simulink model "A5Q3"  (R2017a)
settings: Solver=VariableStepAuto  StartTime=0.0  StopTime=300  MaxStep=0.001  RelTol=1e-3
values from neighbouring files (symbols this model uses):
  alpha_dc = alpha_c/20    (= 0.349219619187)    [Project5Var.m]
  alpha_f = 5*alpha_p    (= 3.49219619187)    [Project5Var.m]
  alpha_fc = 0.5*alpha_c    (= 3.49219619187)    [Project5Var.m]
  C = 1.5*1800/1000*80*10^-6 * Z_base *w_base    (= 1.1558539944)    [Project5Var.m]
  E = 1.0    (= 1)    [Project5Var.m]
  I_base = 1    [Project5Var.m]
  K = sqrt(3/2)    [Project5Var.m]
  ki = alpha_c*(R+Ra)    (= 11.8344493889)    [Project5Var.m]
  ki_dc = alpha_dc^2/2    (= 0.0609771712125)    [Project5Var.m]
  ki_pll = alpha_p^2/2    (= 0.24390868485)    [Project5Var.m]
  kp = alpha_c*Lsigma    (= 1.69441359229)    [Project5Var.m]
  kp_dc = alpha_dc    (= 0.349219619187)    [Project5Var.m]
  kp_pll = alpha_p    (= 0.698439238374)    [Project5Var.m]
  Lsigma = 0.2426    [Project5Var.m]
  Ra = alpha_c*Lsigma-R    (= 1.58785359229)    [Project5Var.m]
  V_base = 1    [Project5Var.m]
  wref = 1.0    (= 1)    [Project5Var.m]
settings Model: Creator=Oskar  LastModifiedBy=Callum

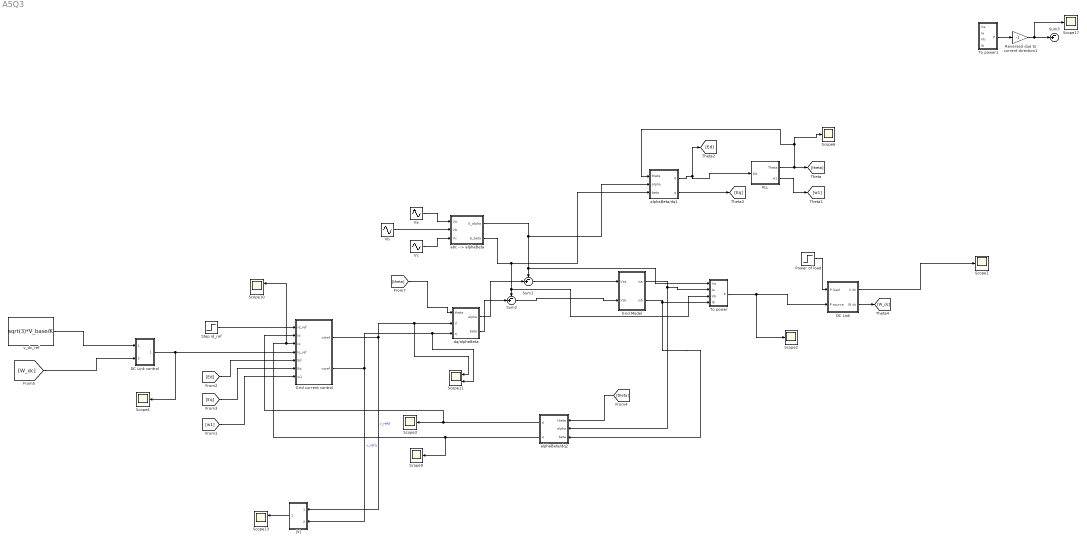
== system A5Q3 ==
  DC Link : Subsystem
  DC Link control : Subsystem
  Grid Model : Subsystem  mask{Ll=Lsigma, Rl=0}
  Grid current control : Subsystem
  PLL : Subsystem
  Power of load : Step  Time=100  Before=0.2  After=0.3  SampleTime=0
  Reversed due to current direction1 : Gain  Gain=-1
  Scope{1..4,6,9,17} (7 alike) : Scope
  Scope10 : Scope  NumInputPorts=2
  Scope11 : Scope  NumInputPorts=2
  Scope13 : Scope  NumInputPorts=2
  Step id_ref : Step  Time=0  After=0  SampleTime=0
  Sum1 : Sum  Inputs=-+|
  Sum2 : Sum  Inputs=-+|
  Sum3 : Sum  Inputs=-+|
  To power : Subsystem
  To power1 : Subsystem
  Va : Sin  Amplitude=E  SampleTime=0
  Vb : Sin  Amplitude=E  Phase=-2*pi/3  SampleTime=0
  Vc : Sin  Amplitude=E  Phase=-4*pi/3  SampleTime=0
  abc --> alphaBeta : Subsystem  mask{K=K}
  alphaBeta/dq1 : Subsystem
  alphaBeta/dq2 : Subsystem
  dq/alphaBeta : Subsystem
  v_dc_ref : Constant  Value=sqrt(3)*V_base/K
  |V| : Subsystem
  wires:
  Va/1 -> abc --> alphaBeta/1(Va)
  abc --> alphaBeta/1(E_alpha) -> To power/1(Va), Sum1/1, alphaBeta/dq1/2(alpha)
  abc --> alphaBeta/2(E_beta) -> alphaBeta/dq1/3("beta "), To power/3(Vb), Sum2/1
  alphaBeta/dq1/2(q) -> [Eq]
  alphaBeta/dq1/1(d) -> PLL/1(Ed), [Ed]
  [theta] -> dq/alphaBeta/1(theta)
  Step id_ref/1 -> Grid current control/1(id_ref)
  Grid current control/1(vdref) -> |V|/1(In1), Scope11/1, dq/alphaBeta/2(d)  "v_refd"
  Grid current control/2(vqref) -> |V|/2(In2), Scope11/2, dq/alphaBeta/3("q ")  "v_refq"
  [Ed] -> Grid current control/5(Ed)
  [Eq] -> Grid current control/6(Eq)
  PLL/2(w1) -> [w1]
  PLL/1(Theta) -> [theta], alphaBeta/dq1/1(theta), Scope6/1
  Vc/1 -> abc --> alphaBeta/3(Vc)
  Vb/1 -> abc --> alphaBeta/2(Vb)
  [theta] -> alphaBeta/dq2/1(theta)
  dq/alphaBeta/1(alpha) -> Sum1/2
  dq/alphaBeta/2(beta) -> Sum2/2
  alphaBeta/dq2/2(q) -> Scope10/1, Grid current control/3(Iq), Scope9/1
  [w1] -> Grid current control/7(w1)
  Sum1/1 -> Grid Model/1(Vsa)
  Grid Model/2(isb) -> To power/4(Ib), alphaBeta/dq2/3("beta ")
  Grid Model/1(isa) -> alphaBeta/dq2/2(alpha), To power/2(Ia)
  Sum2/1 -> Grid Model/2(Vsb)
  ? -> To power1/3(Vb)
  Reversed due to current direction1/1 -> Scope17/1, Sum3/2
  To power1/1(P) -> Reversed due to current direction1/1
  ? -> To power1/4(Ib)
  ? -> To power1/2(Ia)
  ? -> To power1/1(Va)
  alphaBeta/dq2/1(d) -> Grid current control/2(Id), Scope3/1
  v_dc_ref/1 -> DC Link control/1(v_dc ref)
  [W_dc] -> DC Link control/2(W_dc)
  |V|/1(Out1) -> Scope13/1
  DC Link/1(V dc) -> Scope1/1
  DC Link/2(W dc) -> [W_dc]
  To power/1(P) -> Scope2/1, DC Link/2(P source)
  Power of load/1 -> DC Link/1(P load)
  DC Link control/1(iq_ref) -> Scope4/1, Grid current control/4(Iq_ref)

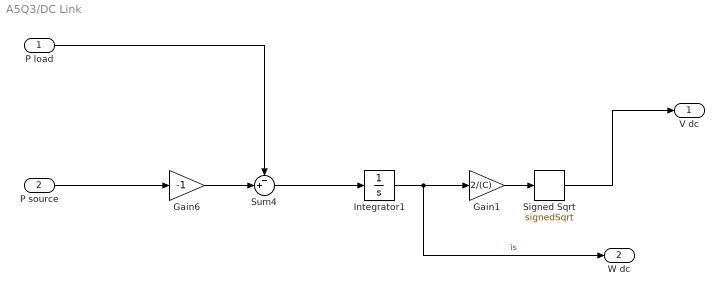
== system A5Q3/DC Link ==
  P load : Inport
  P source : Inport  Port=2
  Gain1 : Gain  Gain=2/(C)
  Gain6 : Gain  Gain=-1
  Integrator1 : Integrator  UpperSaturationLimit=10  LowerSaturationLimit=0
  Signed Sqrt : Sqrt  Operator=signedSqrt  SaturateOnIntegerOverflow=on
  Sum4 : Sum  Inputs=-+|
  V dc : Outport
  W dc : Outport  Port=2
  wires:
  Gain6/1 -> Sum4/2
  P source/1 -> Gain6/1
  P load/1 -> Sum4/1
  Integrator1/1 -> W dc/1, Gain1/1  "is"
  Sum4/1 -> Integrator1/1
  Signed Sqrt/1 -> V dc/1
  Gain1/1 -> Signed Sqrt/1

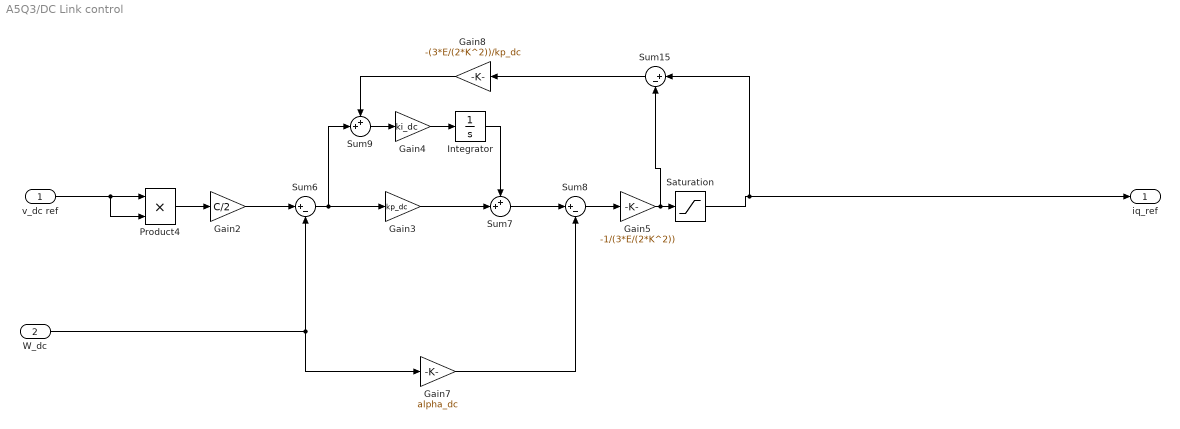
== system A5Q3/DC Link control ==
  v_dc ref : Inport
  W_dc : Inport  Port=2
  Gain2 : Gain  Gain=C/2
  Gain3 : Gain  Gain=kp_dc
  Gain4 : Gain  Gain=ki_dc
  Gain5 : Gain  Gain=-1/(3*E/(2*K^2))
  Gain7 : Gain  Gain=alpha_dc
  Gain8 : Gain  Gain=-(3*E/(2*K^2))/kp_dc
  Integrator : Integrator
  Product4 : Product
  Saturation : Saturate  UpperLimit=I_base  LowerLimit=-I_base
  Sum15 : Sum  Inputs=|+-
  Sum6 : Sum  Inputs=|+-
  Sum7 : Sum  Inputs=++|
  Sum8 : Sum  Inputs=|+-
  Sum9 : Sum  Inputs=++|
  iq_ref : Outport
  wires:
  Gain5/1 -> Sum15/2, Saturation/1
  Gain3/1 -> Sum7/2
  Sum15/1 -> Gain8/1
  Integrator/1 -> Sum7/1
  v_dc ref/1 -> Product4/2, Product4/1
  Product4/1 -> Gain2/1
  Sum7/1 -> Sum8/1
  Gain4/1 -> Integrator/1
  Sum6/1 -> Gain3/1, Sum9/2
  Gain2/1 -> Sum6/1
  Sum8/1 -> Gain5/1
  Saturation/1 -> iq_ref/1, Sum15/1
  Gain7/1 -> Sum8/2
  Sum9/1 -> Gain4/1
  Gain8/1 -> Sum9/1
  W_dc/1 -> Gain7/1, Sum6/2

== system A5Q3/Grid Model ==
  Vsa : Inport
  Vsb : Inport  Port=2
  1/Ll : Gain  Gain=1/Ll
  1/Ll1 : Gain  Gain=1/Ll
  Integrator1 : Integrator
  Integrator2 : Integrator  InitialCondition=-1
  isa : Outport
  isb : Outport  Port=2
  wires:
  Vsa/1 -> 1/Ll/1
  Integrator1/1 -> isa/1  "is"
  1/Ll/1 -> Integrator1/1
  Integrator2/1 -> isb/1  "is"
  1/Ll1/1 -> Integrator2/1
  Vsb/1 -> 1/Ll1/1

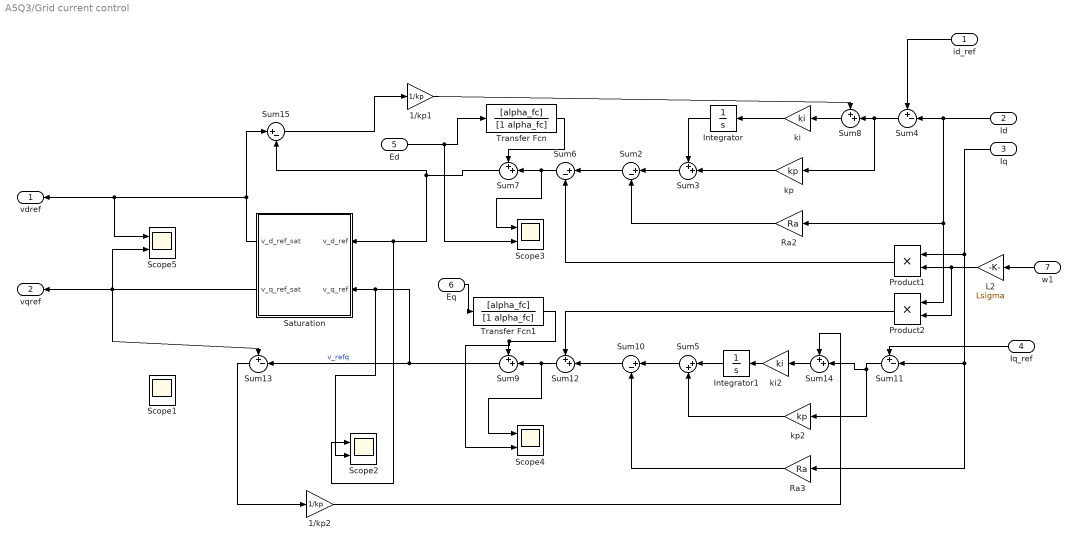
== system A5Q3/Grid current control ==
  id_ref : Inport
  Id : Inport  Port=2
  Iq : Inport  Port=3
  Iq_ref : Inport  Port=4
  Ed : Inport  Port=5
  Eq : Inport  Port=6
  w1 : Inport  Port=7
  1/kp1 : Gain  Gain=1/kp
  1/kp2 : Gain  Gain=1/kp
  Integrator : Integrator
  Integrator1 : Integrator
  L2 : Gain  Gain=Lsigma
  Product1 : Product
  Product2 : Product
  Ra2 : Gain  Gain=Ra
  Ra3 : Gain  Gain=Ra
  Saturation : Subsystem
  Scope1 : Scope
  Scope{2..5} (4 alike) : Scope  NumInputPorts=2
  Sum{2,6,10,15} (4 alike) : Sum  Inputs=|+-
  Sum11 : Sum  Inputs=+-|
  Sum{3,7..9,12,14} (6 alike) : Sum  Inputs=++|
  Sum13 : Sum  Inputs=+-|
  Sum4 : Sum  Inputs=+-|
  Sum5 : Sum  Inputs=|++
  Transfer Fcn : TransferFcn  Numerator=[alpha_fc]  Denominator=[1 alpha_fc]
  Transfer Fcn1 : TransferFcn  Numerator=[alpha_fc]  Denominator=[1 alpha_fc]
  ki : Gain  Gain=ki
  ki2 : Gain  Gain=ki
  kp : Gain  Gain=kp
  kp2 : Gain  Gain=kp
  vdref : Outport
  vqref : Outport  Port=2
  wires:
  Ra2/1 -> Sum2/2
  1/kp2/1 -> Sum14/1
  Sum11/1 -> Sum14/2, kp2/1
  w1/1 -> L2/1
  Sum6/1 -> Scope3/1, Sum7/2
  Ra3/1 -> Sum10/2
  Sum15/1 -> 1/kp1/1
  kp/1 -> Sum3/2
  Sum8/1 -> ki/1
  Sum4/1 -> Sum8/2, kp/1
  Id/1 -> Product2/1, Ra2/1, Sum4/2
  id_ref/1 -> Sum4/1
  Integrator/1 -> Sum3/1
  ki/1 -> Integrator/1
  Sum5/1 -> Sum10/1
  Sum10/1 -> Sum12/2
  Iq_ref/1 -> Sum11/1
  Integrator1/1 -> Sum5/1
  Sum7/1 -> Scope2/1, Saturation/1(v_d_ref), Sum15/2
  Product1/1 -> Sum6/2
  Sum2/1 -> Sum6/1
  Sum3/1 -> Sum2/1
  L2/1 -> Product2/2, Product1/2
  Iq/1 -> Ra3/1, Sum11/2, Product1/1
  Sum14/1 -> ki2/1
  Sum13/1 -> 1/kp2/1
  kp2/1 -> Sum5/2
  Product2/1 -> Sum12/1
  ki2/1 -> Integrator1/1
  1/kp1/1 -> Sum8/1
  Ed/1 -> Scope3/2, Transfer Fcn/1
  Transfer Fcn/1 -> Sum7/1
  Eq/1 -> Transfer Fcn1/1
  Sum9/1 -> Scope2/2, Saturation/2(v_q_ref), Sum13/2  "v_refq"
  Transfer Fcn1/1 -> Scope4/2, Sum9/1
  Sum12/1 -> Scope4/1, Sum9/2
  Saturation/1(v_d_ref_sat) -> Sum15/1, vdref/1, Scope5/1
  Saturation/2(v_q_ref_sat) -> Scope5/2, vqref/1, Sum13/1

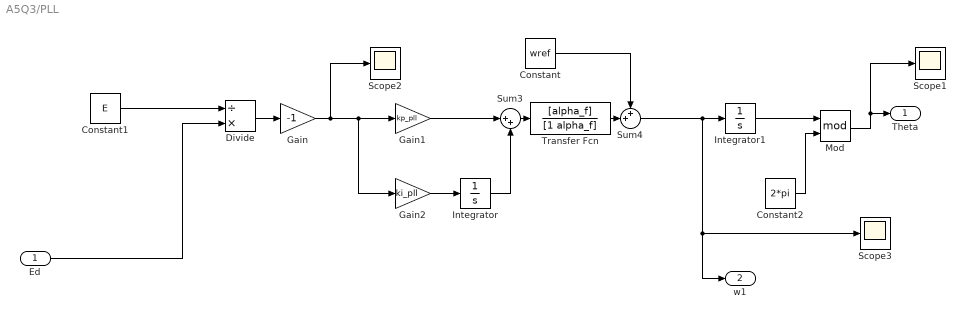
== system A5Q3/PLL ==
  Ed : Inport
  Constant : Constant  Value=wref
  Constant1 : Constant  Value=E
  Constant2 : Constant  Value=2*pi
  Divide : Product  Inputs=/*
  Gain : Gain  Gain=-1
  Gain1 : Gain  Gain=kp_pll
  Gain2 : Gain  Gain=ki_pll
  Integrator : Integrator
  Integrator1 : Integrator
  Mod : Math  Operator=mod  SaturateOnIntegerOverflow=on
  Scope1 : Scope
  Scope2 : Scope
  Scope3 : Scope
  Sum3 : Sum  Inputs=|++
  Sum4 : Sum  Inputs=++|
  Transfer Fcn : TransferFcn  Numerator=[alpha_f]  Denominator=[1 alpha_f]
  Theta : Outport
  w1 : Outport  Port=2
  wires:
  Gain/1 -> Scope2/1, Gain1/1, Gain2/1
  Ed/1 -> Divide/2
  Gain1/1 -> Sum3/1
  Divide/1 -> Gain/1
  Gain2/1 -> Integrator/1
  Constant1/1 -> Divide/1
  Constant2/1 -> Mod/2
  Integrator1/1 -> Mod/1
  Integrator/1 -> Sum3/2
  Mod/1 -> Scope1/1, Theta/1
  Constant/1 -> Sum4/1
  Sum4/1 -> Scope3/1, w1/1, Integrator1/1
  Sum3/1 -> Transfer Fcn/1
  Transfer Fcn/1 -> Sum4/2

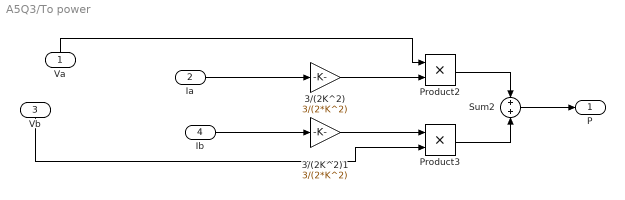
== system A5Q3/To power ==
  Va : Inport
  Ia : Inport  Port=2
  Vb : Inport  Port=3
  Ib : Inport  Port=4
  3/(2K^2) : Gain  Gain=3/(2*K^2)
  3/(2K^2)1 : Gain  Gain=3/(2*K^2)
  Product2 : Product
  Product3 : Product
  Sum2 : Sum
  P : Outport
  wires:
  3/(2K^2)1/1 -> Product3/1
  3/(2K^2)/1 -> Product2/2
  Product2/1 -> Sum2/1
  Ia/1 -> 3/(2K^2)/1
  Vb/1 -> Product3/2
  Va/1 -> Product2/1
  Ib/1 -> 3/(2K^2)1/1
  Product3/1 -> Sum2/2
  Sum2/1 -> P/1

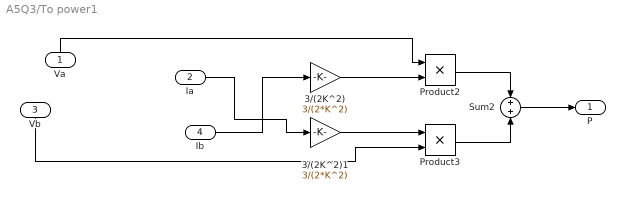
== system A5Q3/To power1 ==
  Va : Inport
  Ia : Inport  Port=2
  Vb : Inport  Port=3
  Ib : Inport  Port=4
  3/(2K^2) : Gain  Gain=3/(2*K^2)
  3/(2K^2)1 : Gain  Gain=3/(2*K^2)
  Product2 : Product
  Product3 : Product
  Sum2 : Sum
  P : Outport
  wires:
  3/(2K^2)1/1 -> Product3/1
  3/(2K^2)/1 -> Product2/2
  Product2/1 -> Sum2/1
  Vb/1 -> Product3/2
  Va/1 -> Product2/1
  Product3/1 -> Sum2/2
  Sum2/1 -> P/1
  Ib/1 -> 3/(2K^2)/1
  Ia/1 -> 3/(2K^2)1/1

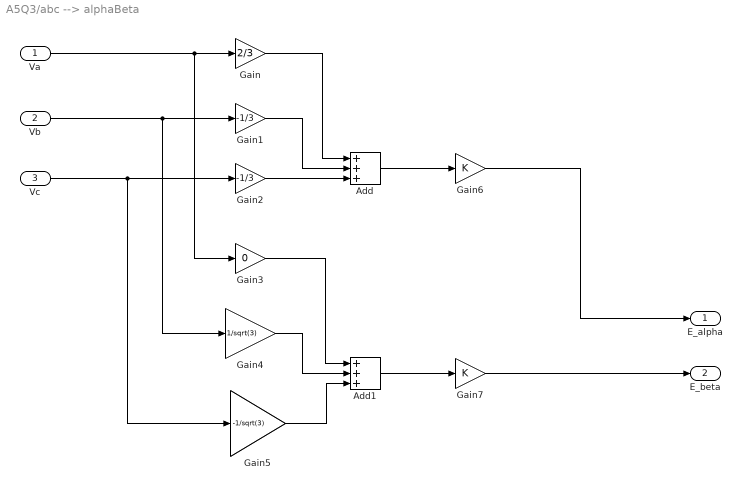
== system A5Q3/abc --> alphaBeta ==
  Va : Inport
  Vb : Inport  Port=2
  Vc : Inport  Port=3
  Add : Sum  Inputs=+++
  Add1 : Sum  Inputs=+++
  Gain : Gain  Gain=2/3
  Gain1 : Gain  Gain=-1/3
  Gain2 : Gain  Gain=-1/3
  Gain3 : Gain  Gain=0
  Gain4 : Gain  Gain=1/sqrt(3)
  Gain5 : Gain  Gain=-1/sqrt(3)
  Gain6 : Gain  Gain=K
  Gain7 : Gain  Gain=K
  E_alpha : Outport
  E_beta : Outport  Port=2
  wires:
  Add/1 -> Gain6/1
  Va/1 -> Gain3/1, Gain/1
  Vc/1 -> Gain5/1, Gain2/1
  Vb/1 -> Gain4/1, Gain1/1
  Gain3/1 -> Add1/1
  Gain6/1 -> E_alpha/1
  Gain7/1 -> E_beta/1
  Add1/1 -> Gain7/1
  Gain1/1 -> Add/2
  Gain/1 -> Add/1
  Gain5/1 -> Add1/3
  Gain2/1 -> Add/3
  Gain4/1 -> Add1/2

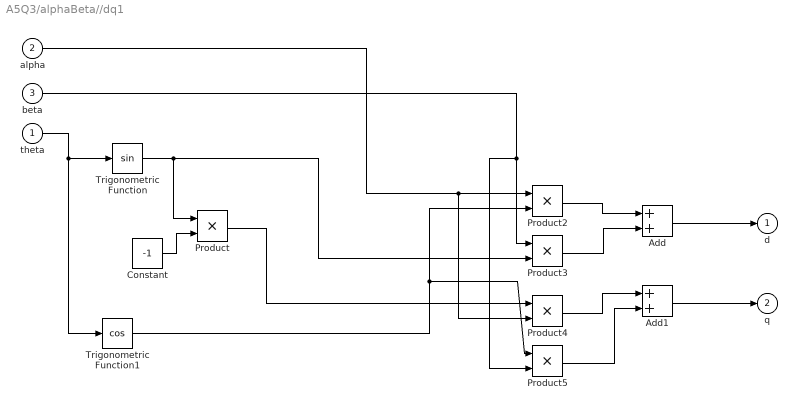
== system A5Q3/alphaBeta//dq1 ==
  theta : Inport
  alpha : Inport  Port=2
  "beta " : Inport  Port=3
  Add : Sum
  Add1 : Sum
  Constant : Constant  Value=-1
  Product{,2..5} (5 alike) : Product
  Trigonometric Function : Trigonometry
  Trigonometric Function1 : Trigonometry  Operator=cos
  d : Outport
  q : Outport  Port=2
  wires:
  theta/1 -> Trigonometric Function1/1, Trigonometric Function/1
  Product4/1 -> Add1/1
  Product5/1 -> Add1/2
  Trigonometric Function1/1 -> Product2/2, Product5/1
  Product/1 -> Product4/1
  Trigonometric Function/1 -> Product/1, Product3/2
  Add1/1 -> q/1
  alpha/1 -> Product2/1, Product4/2
  "beta "/1 -> Product5/2, Product3/1
  Add/1 -> d/1
  Constant/1 -> Product/2
  Product2/1 -> Add/1
  Product3/1 -> Add/2

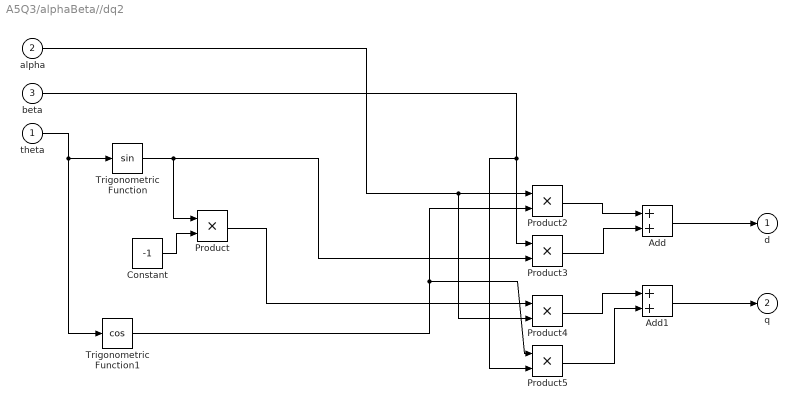
== system A5Q3/alphaBeta//dq2 ==
  theta : Inport
  alpha : Inport  Port=2
  "beta " : Inport  Port=3
  Add : Sum
  Add1 : Sum
  Constant : Constant  Value=-1
  Product{,2..5} (5 alike) : Product
  Trigonometric Function : Trigonometry
  Trigonometric Function1 : Trigonometry  Operator=cos
  d : Outport
  q : Outport  Port=2
  wires:
  theta/1 -> Trigonometric Function1/1, Trigonometric Function/1
  Product4/1 -> Add1/1
  Product5/1 -> Add1/2
  Trigonometric Function1/1 -> Product2/2, Product5/1
  Product/1 -> Product4/1
  Trigonometric Function/1 -> Product/1, Product3/2
  Add1/1 -> q/1
  alpha/1 -> Product2/1, Product4/2
  "beta "/1 -> Product5/2, Product3/1
  Add/1 -> d/1
  Constant/1 -> Product/2
  Product2/1 -> Add/1
  Product3/1 -> Add/2

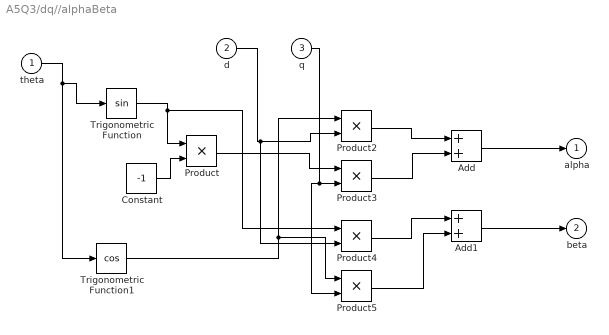
== system A5Q3/dq//alphaBeta ==
  theta : Inport
  d : Inport  Port=2
  "q " : Inport  Port=3
  Add : Sum
  Add1 : Sum
  Constant : Constant  Value=-1
  Product{,2..5} (5 alike) : Product
  Trigonometric Function : Trigonometry
  Trigonometric Function1 : Trigonometry  Operator=cos
  alpha : Outport
  beta : Outport  Port=2
  wires:
  theta/1 -> Trigonometric Function1/1, Trigonometric Function/1
  Product4/1 -> Add1/1
  Product5/1 -> Add1/2
  Trigonometric Function/1 -> Product4/1, Product/1
  Add1/1 -> beta/1
  Add/1 -> alpha/1
  Constant/1 -> Product/2
  Product2/1 -> Add/1
  Product3/1 -> Add/2
  Trigonometric Function1/1 -> Product5/1, Product2/1
  Product/1 -> Product3/1
  d/1 -> Product4/2, Product2/2
  "q "/1 -> Product3/2, Product5/2

== system A5Q3/|V| ==
  In1 : Inport
  In2 : Inport  Port=2
  Product1 : Product
  Product2 : Product
  Sqrt : Sqrt  SaturateOnIntegerOverflow=on
  Sum : Sum  Inputs=|++
  Out1 : Outport
  wires:
  Product1/1 -> Sum/1
  Product2/1 -> Sum/2
  Sqrt/1 -> Out1/1
  Sum/1 -> Sqrt/1
  In2/1 -> Product1/1, Product1/2
  In1/1 -> Product2/2, Product2/1

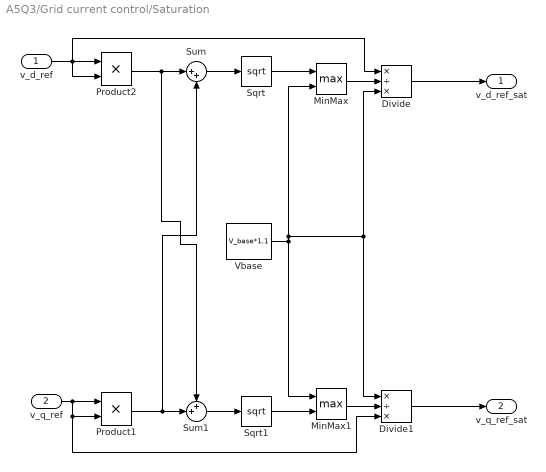
== system A5Q3/Grid current control/Saturation ==
  v_d_ref : Inport
  v_q_ref : Inport  Port=2
  Divide : Product  Inputs=*/*
  Divide1 : Product  Inputs=*/*
  MinMax : MinMax  Function=max  Inputs=2
  MinMax1 : MinMax  Function=max  Inputs=2
  Product1 : Product
  Product2 : Product
  Sqrt : Sqrt  SaturateOnIntegerOverflow=on
  Sqrt1 : Sqrt  SaturateOnIntegerOverflow=on
  Sum : Sum  Inputs=|++
  Sum1 : Sum  Inputs=++|
  Vbase : Constant  Value=V_base*1.1
  v_d_ref_sat : Outport
  v_q_ref_sat : Outport  Port=2
  wires:
  Sum1/1 -> Sqrt1/1
  MinMax1/1 -> Divide1/2
  Sum/1 -> Sqrt/1
  Product2/1 -> Sum/1, Sum1/1
  MinMax/1 -> Divide/2
  Sqrt1/1 -> MinMax1/2
  Vbase/1 -> MinMax/2, Divide/3, Divide1/1, MinMax1/1
  Divide/1 -> v_d_ref_sat/1
  Divide1/1 -> v_q_ref_sat/1
  Product1/1 -> Sum/2, Sum1/2
  Sqrt/1 -> MinMax/1
  v_d_ref/1 -> Divide/1, Product2/2, Product2/1
  v_q_ref/1 -> Divide1/3, Product1/2, Product1/1
